simulink model "fuzzy"  (Simulink 8.4)
settings: Solver=ode45  StartTime=0.0  StopTime=20  RelTol=1e-8  AbsTol=1e-8
values from neighbouring files (symbols this model uses):
  A1 = [0 0 1 0; 0 0 0 1; 0 i j 0; 0 k l 0]    [data.m]
  A2 = [0 0 1 0; 0 0 0 1; 0 i2 j2 0; 0 k2 l2 0]    [data.m]
  A3 = [0 0 1 0; 0 0 0 1; 0 i3 j3 0; 0 k3 l3 0]    [data.m]
  A4 = [0 0 1 0; 0 0 0 1; 0 i4 j4 0; 0 k4 l4 0]    [data.m]
  A5 = [0 0 1 0; 0 0 0 1; 0 i5 j5 0; 0 k5 l5 0]    [data.m]
  A6 = [0 0 1 0; 0 0 0 1; 0 i6 j6 0; 0 k6 l6 0]    [data.m]
  A7 = [0 0 1 0; 0 0 0 1; 0 i7 j7 0; 0 k7 l7 0]    [data.m]
  A8 = [0 0 1 0; 0 0 0 1; 0 i8 j8 0; 0 k8 l8 0]    [data.m]
  A9 = [0 0 1 0; 0 0 0 1; 0 i9 j9 0; 0 k9 l9 0]    [data.m]
  B1 = [0; 0; n; o]    [data.m]
  B2 = [0; 0; n2; o2]    [data.m]
  B3 = [0; 0; n3; o3]    [data.m]
  B4 = [0; 0; n4; o4]    [data.m]
  B5 = [0; 0; n5; o5]    [data.m]
  B6 = [0; 0; n6; o6]    [data.m]
  B7 = [0; 0; n7; o7]    [data.m]
  B8 = [0; 0; n8; o8]    [data.m]
  B9 = [0; 0; n9; o9]    [data.m]
  B_eq = 0    [data.m]
  g = 9.81    [data.m]
  initial = pi/2    (= 1.57079632679)    [data.m]
  J_eq = 1.23e-4    (= 0.000123)    [data.m]
  J_p = 1.20e-4    (= 0.00012)    [data.m]
  K_m = K_t    (= 0.028)    [data.m]
  K_t = 0.028    [data.m]
  K_w = 2.3    [data.m]
  l_p = 0.191    [data.m]
  m = 0.027    [data.m]
  r = 0.0826    [data.m]
  R_m = 3.3    [data.m]
libraries: fuzblock x9
settings Model: Creator=Crush  LastModifiedBy=Aramil_2

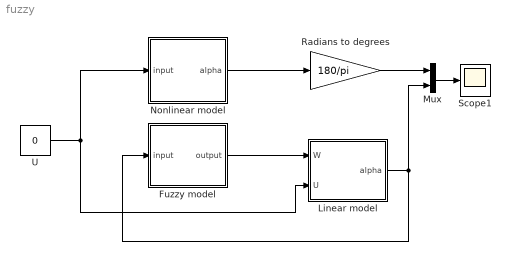
== system fuzzy ==
  Fuzzy model : Subsystem
  Linear model : Subsystem
  Mux : Mux  Inputs=2
  Nonlinear model : Subsystem
  Radians to degrees : Gain  Gain=180/pi
  Scope1 : Scope
      settings: YMin=167.5  YMax=195
  U : Constant  Value=0
  wires:
  Nonlinear model/1(alpha) -> Radians to degrees/1
  Radians to degrees/1 -> Mux/1
  Mux/1 -> Scope1/1
  Linear model/1(alpha) -> Fuzzy model/1(input), Mux/2
  Fuzzy model/1(output) -> Linear model/1(W)
  U/1 -> Linear model/2(U), Nonlinear model/1(input)

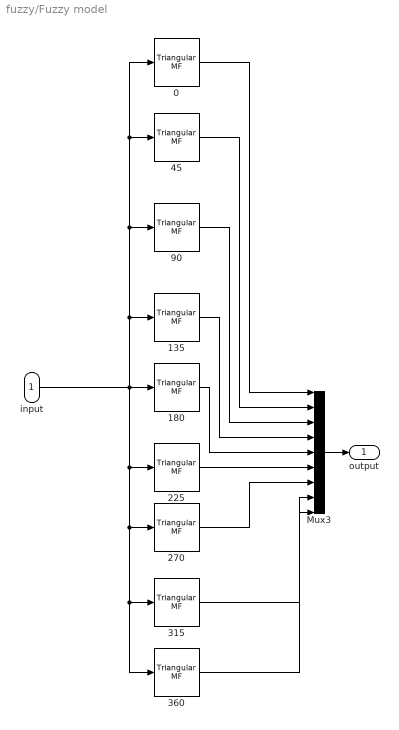
== system fuzzy/Fuzzy model ==
  input : Inport
  0 : fuzblock/Membership  Functions/Triangular MF  a=0  b=0  c=90
  135 : fuzblock/Membership  Functions/Triangular MF  a=90  b=135  c=180
  180 : fuzblock/Membership  Functions/Triangular MF  a=130  b=180  c=225
  225 : fuzblock/Membership  Functions/Triangular MF  a=180  b=225  c=270
  270 : fuzblock/Membership  Functions/Triangular MF  a=225  b=270  c=315
  315 : fuzblock/Membership  Functions/Triangular MF  a=280  b=315  c=360
  360 : fuzblock/Membership  Functions/Triangular MF  a=270  b=360  c=360
  45 : fuzblock/Membership  Functions/Triangular MF  a=0  b=45  c=90
  90 : fuzblock/Membership  Functions/Triangular MF  a=45  b=90  c=130
  Mux3 : Mux  Inputs=9
  output : Outport
  wires:
  Mux3/1 -> output/1
  input/1 -> 360/1, 315/1, 270/1, 225/1, 135/1, 45/1, 0/1, 90/1, 180/1
  360/1 -> Mux3/9
  315/1 -> Mux3/8
  270/1 -> Mux3/7
  225/1 -> Mux3/6
  180/1 -> Mux3/5
  135/1 -> Mux3/4
  90/1 -> Mux3/3
  45/1 -> Mux3/2
  0/1 -> Mux3/1

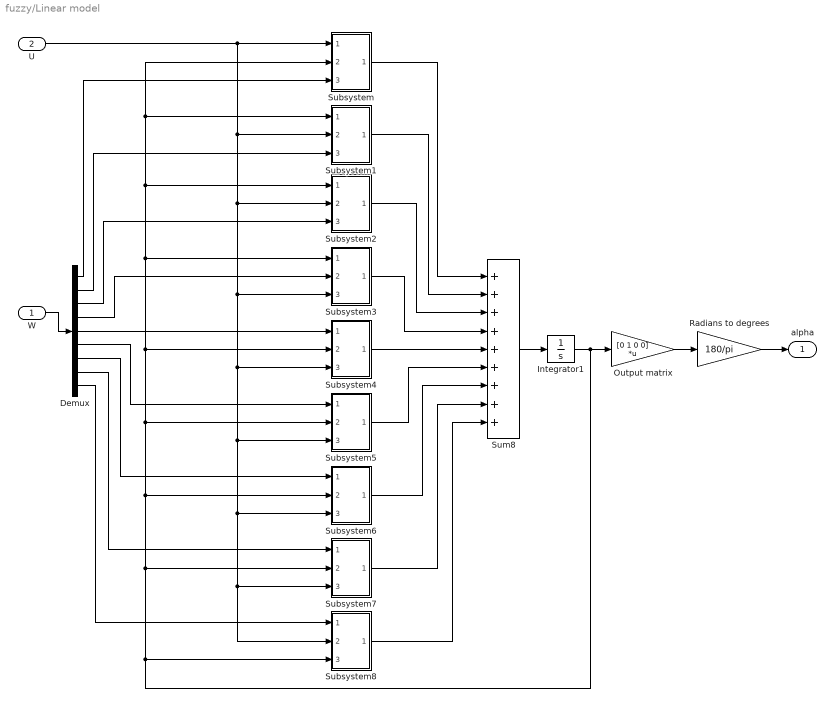
== system fuzzy/Linear model ==
  W : Inport
  U : Inport  Port=2
  Demux : Demux  Outputs=9
  Integrator1 : Integrator  InitialCondition=|  UpperSaturationLimit=3.14  LowerSaturationLimit=-3.14
      | [0;             initial
      | 
      | 
      | 
      | 
      | 
      | 
      | 
      | 
      | ;  0; 0]
  Output matrix : Gain  Gain=[0 1 0 0]  Multiplication=Matrix(K*u)
  Radians to degrees : Gain  Gain=180/pi
  Subsystem : Subsystem
  Subsystem1 : Subsystem
  Subsystem2 : Subsystem
  Subsystem3 : Subsystem
  Subsystem4 : Subsystem
  Subsystem5 : Subsystem
  Subsystem6 : Subsystem
  Subsystem7 : Subsystem
  Subsystem8 : Subsystem
  Sum8 : Sum  Inputs=+++++++++
  alpha : Outport
  wires:
  Output matrix/1 -> Radians to degrees/1
  W/1 -> Demux/1
  Radians to degrees/1 -> alpha/1
  Sum8/1 -> Integrator1/1
  Integrator1/1 -> Subsystem3/1(In1), Subsystem2/1(In1), Subsystem/2(In2), Subsystem1/1(In1), Subsystem4/2(In2), Subsystem5/2(In2), Subsystem6/2(In2), Subsystem7/2(In2), Subsystem8/3(In3), Output matrix/1
  U/1 -> Subsystem/1(In1), Subsystem8/2(In2), Subsystem7/3(In3), Subsystem6/3(In3), Subsystem5/3(In3), Subsystem4/3(In3), Subsystem3/3(In3), Subsystem2/2(In2), Subsystem1/2(In2)
  Demux/1 -> Subsystem/3(In3)
  Subsystem/1(Out1) -> Sum8/1
  Demux/2 -> Subsystem1/3(In3)
  Subsystem1/1(Out1) -> Sum8/2
  Demux/3 -> Subsystem2/3(In3)
  Subsystem2/1(Out1) -> Sum8/3
  Demux/4 -> Subsystem3/2(In2)
  Subsystem3/1(Out1) -> Sum8/4
  Demux/5 -> Subsystem4/1(In1)
  Subsystem4/1(Out1) -> Sum8/5
  Demux/6 -> Subsystem5/1(In1)
  Subsystem5/1(Out1) -> Sum8/6
  Demux/7 -> Subsystem6/1(In1)
  Subsystem6/1(Out1) -> Sum8/7
  Demux/8 -> Subsystem7/1(In1)
  Subsystem7/1(Out1) -> Sum8/8
  Demux/9 -> Subsystem8/1(In1)
  Subsystem8/1(Out1) -> Sum8/9

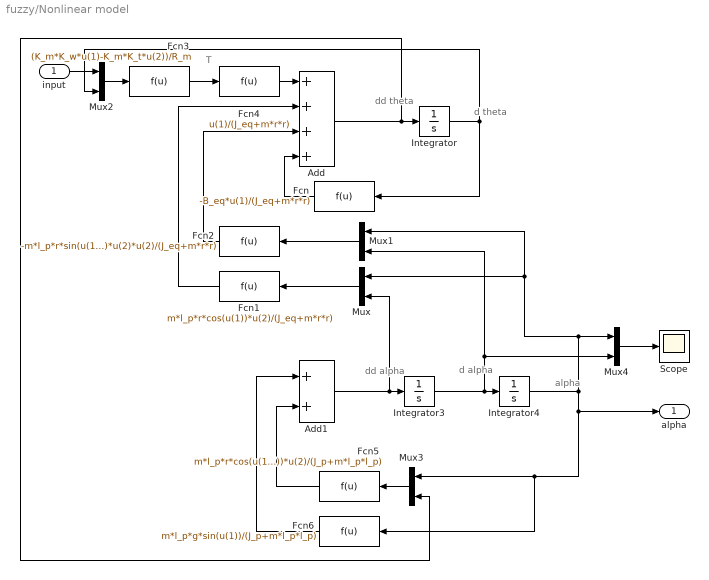
== system fuzzy/Nonlinear model ==
  note: dd theta
  note: d theta
  note: dd alpha
  note: d alpha
  note: alpha
  note: T
  input : Inport
  Add : Sum  Inputs=++++
  Add1 : Sum
  Fcn : Fcn  Expr=-B_eq*u(1)/(J_eq+m*r*r)
  Fcn1 : Fcn  Expr=m*l_p*r*cos(u(1))*u(2)/(J_eq+m*r*r)
  Fcn2 : Fcn  Expr=-m*l_p*r*sin(u(1))*u(2)*u(2)/(J_eq+m*r*r)
  Fcn3 : Fcn  Expr=(K_m*K_w*u(1)-K_m*K_t*u(2))/R_m
  Fcn4 : Fcn  Expr=u(1)/(J_eq+m*r*r)
  Fcn5 : Fcn  Expr=m*l_p*r*cos(u(1))*u(2)/(J_p+m*l_p*l_p)
  Fcn6 : Fcn  Expr=m*l_p*g*sin(u(1))/(J_p+m*l_p*l_p)
  Integrator : Integrator
  Integrator3 : Integrator
  Integrator4 : Integrator  InitialCondition=initial
  Mux{,1..4} (5 alike) : Mux  Inputs=2
  Scope : Scope
      settings: SaveName=ScopeData7
  alpha : Outport
  wires:
  Add/1 -> Integrator/1, Mux3/2
  Integrator/1 -> Fcn/1, Mux2/2
  Add1/1 -> Integrator3/1, Mux/2
  Integrator3/1 -> Integrator4/1, Mux4/2, Mux1/2
  Integrator4/1 -> Fcn6/1, Mux3/1, alpha/1, Mux/1, Mux1/1, Mux4/1
  Mux/1 -> Fcn1/1
  Mux1/1 -> Fcn2/1
  Mux2/1 -> Fcn3/1
  Fcn3/1 -> Fcn4/1
  Fcn4/1 -> Add/1
  Fcn/1 -> Add/4
  Fcn2/1 -> Add/3
  Fcn1/1 -> Add/2
  Mux3/1 -> Fcn5/1
  Fcn5/1 -> Add1/2
  Fcn6/1 -> Add1/1
  input/1 -> Mux2/1
  Mux4/1 -> Scope/1

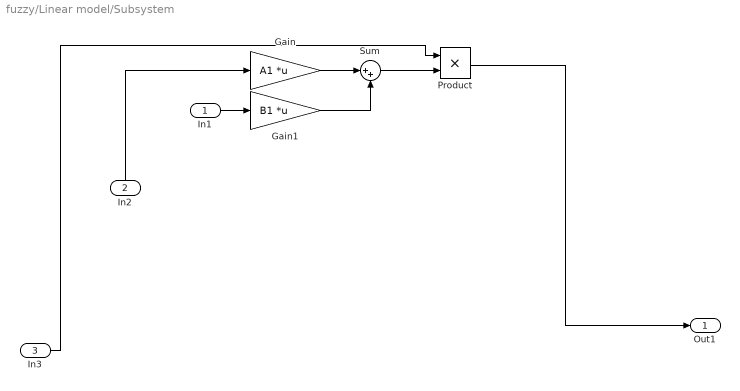
== system fuzzy/Linear model/Subsystem ==
  In1 : Inport
  In2 : Inport  Port=2
  In3 : Inport  Port=3
  Gain : Gain  Gain=A1  Multiplication=Matrix(K*u)
  Gain1 : Gain  Gain=B1  Multiplication=Matrix(K*u)
  Product : Product  RndMeth=Zero
  Sum : Sum  Inputs=|++
  Out1 : Outport
  wires:
  Gain/1 -> Sum/1
  Gain1/1 -> Sum/2
  Product/1 -> Out1/1
  Sum/1 -> Product/2
  In3/1 -> Product/1
  In1/1 -> Gain1/1
  In2/1 -> Gain/1

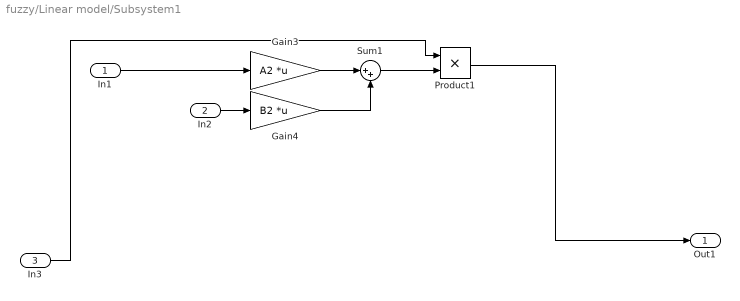
== system fuzzy/Linear model/Subsystem1 ==
  In1 : Inport
  In2 : Inport  Port=2
  In3 : Inport  Port=3
  Gain3 : Gain  Gain=A2  Multiplication=Matrix(K*u)
  Gain4 : Gain  Gain=B2  Multiplication=Matrix(K*u)
  Product1 : Product  RndMeth=Zero
  Sum1 : Sum  Inputs=|++
  Out1 : Outport
  wires:
  Gain4/1 -> Sum1/2
  Gain3/1 -> Sum1/1
  Product1/1 -> Out1/1
  Sum1/1 -> Product1/2
  In3/1 -> Product1/1
  In2/1 -> Gain4/1
  In1/1 -> Gain3/1

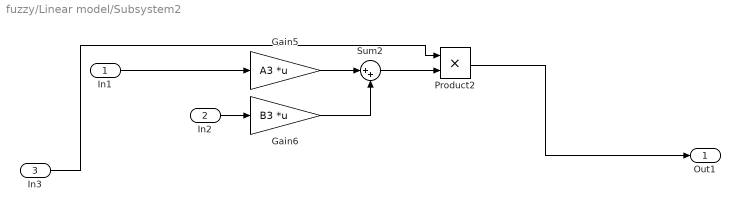
== system fuzzy/Linear model/Subsystem2 ==
  In1 : Inport
  In2 : Inport  Port=2
  In3 : Inport  Port=3
  Gain5 : Gain  Gain=A3  Multiplication=Matrix(K*u)
  Gain6 : Gain  Gain=B3  Multiplication=Matrix(K*u)
  Product2 : Product  RndMeth=Zero
  Sum2 : Sum  Inputs=|++
  Out1 : Outport
  wires:
  Gain5/1 -> Sum2/1
  Gain6/1 -> Sum2/2
  Product2/1 -> Out1/1
  Sum2/1 -> Product2/2
  In2/1 -> Gain6/1
  In1/1 -> Gain5/1
  In3/1 -> Product2/1

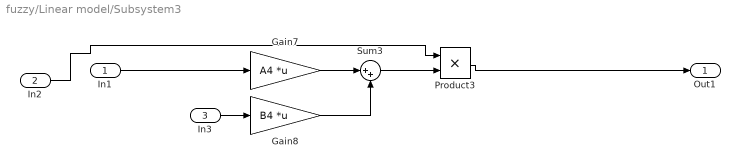
== system fuzzy/Linear model/Subsystem3 ==
  In1 : Inport
  In2 : Inport  Port=2
  In3 : Inport  Port=3
  Gain7 : Gain  Gain=A4  Multiplication=Matrix(K*u)
  Gain8 : Gain  Gain=B4  Multiplication=Matrix(K*u)
  Product3 : Product  RndMeth=Zero
  Sum3 : Sum  Inputs=|++
  Out1 : Outport
  wires:
  Gain7/1 -> Sum3/1
  Gain8/1 -> Sum3/2
  Product3/1 -> Out1/1
  Sum3/1 -> Product3/2
  In2/1 -> Product3/1
  In3/1 -> Gain8/1
  In1/1 -> Gain7/1

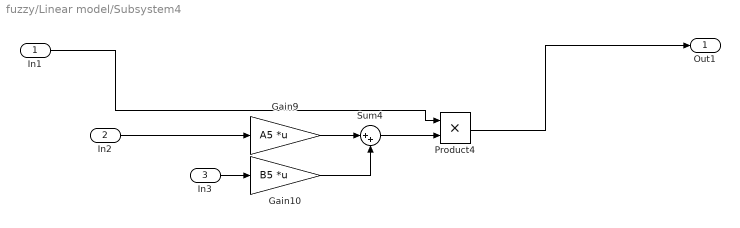
== system fuzzy/Linear model/Subsystem4 ==
  In1 : Inport
  In2 : Inport  Port=2
  In3 : Inport  Port=3
  Gain10 : Gain  Gain=B5  Multiplication=Matrix(K*u)
  Gain9 : Gain  Gain=A5  Multiplication=Matrix(K*u)
  Product4 : Product  RndMeth=Zero
  Sum4 : Sum  Inputs=|++
  Out1 : Outport
  wires:
  Gain10/1 -> Sum4/2
  Gain9/1 -> Sum4/1
  Product4/1 -> Out1/1
  Sum4/1 -> Product4/2
  In1/1 -> Product4/1
  In3/1 -> Gain10/1
  In2/1 -> Gain9/1

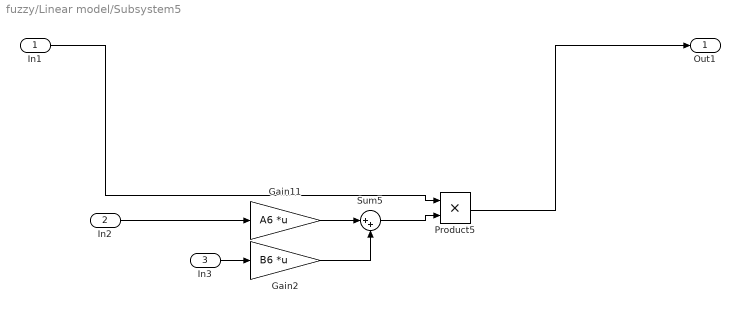
== system fuzzy/Linear model/Subsystem5 ==
  In1 : Inport
  In2 : Inport  Port=2
  In3 : Inport  Port=3
  Gain11 : Gain  Gain=A6  Multiplication=Matrix(K*u)
  Gain2 : Gain  Gain=B6  Multiplication=Matrix(K*u)
  Product5 : Product  RndMeth=Zero
  Sum5 : Sum  Inputs=|++
  Out1 : Outport
  wires:
  Gain11/1 -> Sum5/1
  Gain2/1 -> Sum5/2
  Product5/1 -> Out1/1
  Sum5/1 -> Product5/2
  In1/1 -> Product5/1
  In3/1 -> Gain2/1
  In2/1 -> Gain11/1

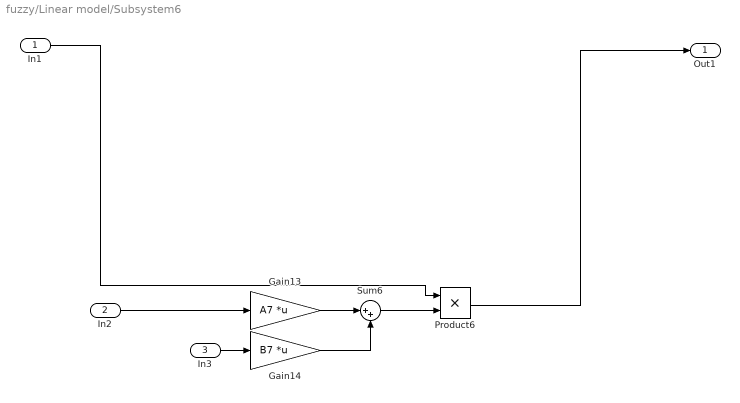
== system fuzzy/Linear model/Subsystem6 ==
  In1 : Inport
  In2 : Inport  Port=2
  In3 : Inport  Port=3
  Gain13 : Gain  Gain=A7  Multiplication=Matrix(K*u)
  Gain14 : Gain  Gain=B7  Multiplication=Matrix(K*u)
  Product6 : Product  RndMeth=Zero
  Sum6 : Sum  Inputs=|++
  Out1 : Outport
  wires:
  Gain13/1 -> Sum6/1
  Gain14/1 -> Sum6/2
  Product6/1 -> Out1/1
  Sum6/1 -> Product6/2
  In1/1 -> Product6/1
  In3/1 -> Gain14/1
  In2/1 -> Gain13/1

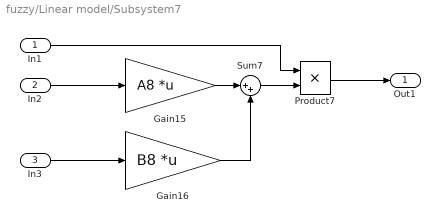
== system fuzzy/Linear model/Subsystem7 ==
  In1 : Inport
  In2 : Inport  Port=2
  In3 : Inport  Port=3
  Gain15 : Gain  Gain=A8  Multiplication=Matrix(K*u)
  Gain16 : Gain  Gain=B8  Multiplication=Matrix(K*u)
  Product7 : Product  RndMeth=Zero
  Sum7 : Sum  Inputs=|++
  Out1 : Outport
  wires:
  Gain15/1 -> Sum7/1
  Gain16/1 -> Sum7/2
  Sum7/1 -> Product7/2
  Product7/1 -> Out1/1
  In1/1 -> Product7/1
  In3/1 -> Gain16/1
  In2/1 -> Gain15/1

== system fuzzy/Linear model/Subsystem8 ==
  In1 : Inport
  In2 : Inport  Port=2
  In3 : Inport  Port=3
  Gain40 : Gain  Gain=A9  Multiplication=Matrix(K*u)
  Gain41 : Gain  Gain=B9  Multiplication=Matrix(K*u)
  Product17 : Product  RndMeth=Zero
  Sum19 : Sum  Inputs=|++
  Out1 : Outport
  wires:
  Gain41/1 -> Sum19/2
  Sum19/1 -> Product17/2
  Gain40/1 -> Sum19/1
  Product17/1 -> Out1/1
  In1/1 -> Product17/1
  In2/1 -> Gain41/1
  In3/1 -> Gain40/1
